simulink model "fir_filter"  (R2025b)
settings: Solver=VariableStepAuto  StartTime=0.0  StopTime=10.0  RelTol=1e-3
undefined symbols (not defined in the file or in its folder): b_coeff, dspblkCoreblockFVToolHelper, gcbh
libraries: hdlsllib x1
settings Model: Creator=strog  LastModifiedBy=strog

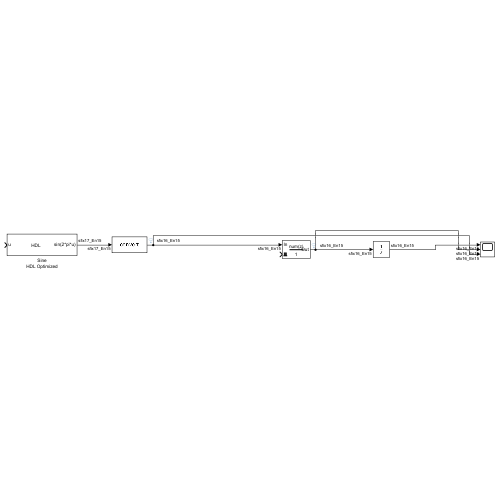
[thumbnail: Simulink's stored preview of the top-level diagram]
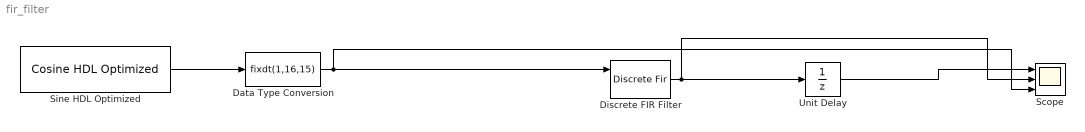
== system fir_filter ==
  Data Type Conversion : DataTypeConversion  OutDataTypeStr=fixdt(1,16,15)  RndMeth=Nearest
  Discrete FIR Filter : DiscreteFir  LoadFcn=dspblkCoreblockFVToolHelper(gcbh,'load');  Coefficients=b_coeff  ExternalReset=Level  CoefDataTypeStr=fixdt(1,16,15)  ProductDataTypeStr=fixdt(1,32,30)  AccumDataTypeStr=fixdt(1,34,30)  OutDataTypeStr=fixdt(1, 16, 15)  RndMeth=Nearest  SaturateOnIntegerOverflow=on
      settings: CopyFcn=dspblkCoreblockFVToolHelper(gcbh,'copy');  DeleteFcn=dspblkCoreblockFVToolHelper(gcbh,'close');  ModelCloseFcn=dspblkCoreblockFVToolHelper(gcbh,'close');  PreSaveFcn=dspblkCoreblockFVToolHelper(gcbh,'presave');  PostSaveFcn=dspblkCoreblockFVToolHelper(gcbh,'postsave');  CloseFcn=dspblkCoreblockFVToolHelper(gcbh,'close');  InputPortMap=u0,r6
  Scope : Scope  NumInputPorts=3
      settings: DataLoggingVariableName=ScopeData2  DataLoggingSaveFormat=Array
  Sine HDL Optimized : hdlsllib/Lookup Tables/Cosine HDL Optimized  OutputFormula=sin(2*pi*u)  NumDataPoints=64  TableDataTypeStr=fixdt(0,16,15)  SimulateLUTROMDelay=off
      settings: LibrarySourceBlock=|
      | hdlsllib/Lookup
      | Tables/Sine
      | HDL Optimized
  Unit Delay : UnitDelay  SampleTime=1e-8  HasFrameUpgradeWarning=on
  wires:
  Discrete FIR Filter/1 -> Scope/2, Unit Delay/1
  Data Type Conversion/1 -> Scope/3, Discrete FIR Filter/1
  Sine HDL Optimized/1 -> Data Type Conversion/1
  Unit Delay/1 -> Scope/1
